simulink model "Ejercicio"  (R2023b)
settings: Solver=VariableStepAuto  StartTime=0.0  StopTime=100  RelTol=1e-3
settings Model: Creator=20808  LastModifiedBy=20808

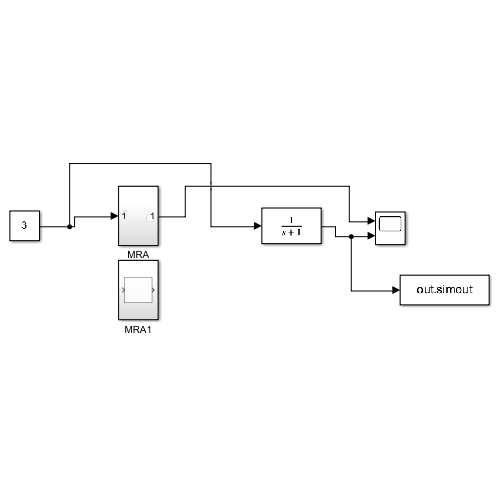
[thumbnail: Simulink's stored preview of the top-level diagram]
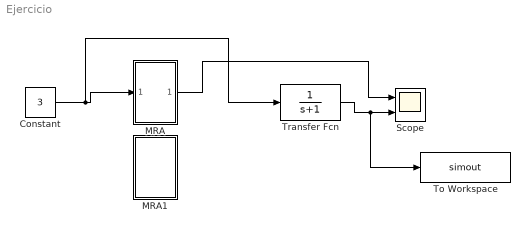
== system Ejercicio ==
  Constant : Constant  Value=3
  MRA : Subsystem
  MRA1 : Subsystem
  Scope : Scope  NumInputPorts=2
  To Workspace : ToWorkspace  VariableName=simout  SampleTime=-1
  Transfer Fcn : TransferFcn  Denominator=[1 1]
  wires:
  Constant/1 -> Transfer Fcn/1, MRA/1(In1)
  MRA/1(Out1) -> Scope/1
  Transfer Fcn/1 -> To Workspace/1, Scope/2

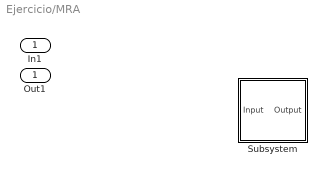
== system Ejercicio/MRA ==
  In1 : Inport
  Subsystem : Subsystem
  Out1 : Outport

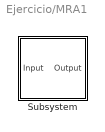
== system Ejercicio/MRA1 ==
  Subsystem : Subsystem

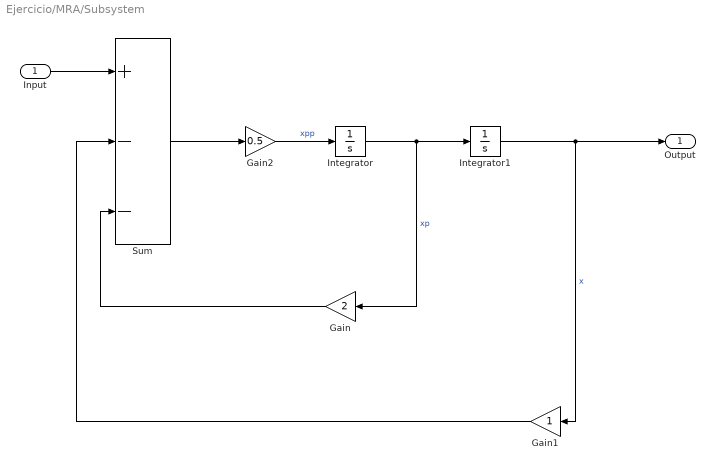
== system Ejercicio/MRA/Subsystem ==
  Input : Inport
  Gain : Gain  Gain=2
  Gain1 : Gain
  Gain2 : Gain  Gain=0.5
  Integrator : Integrator
  Integrator1 : Integrator
  Sum : Sum  Inputs=+--
  Output : Outport
  wires:
  Gain2/1 -> Integrator/1  "xpp"
  Sum/1 -> Gain2/1
  Integrator1/1 -> Output/1, Gain1/1  "x"
  Gain/1 -> Sum/3
  Input/1 -> Sum/1
  Gain1/1 -> Sum/2
  Integrator/1 -> Gain/1, Integrator1/1  "xp"

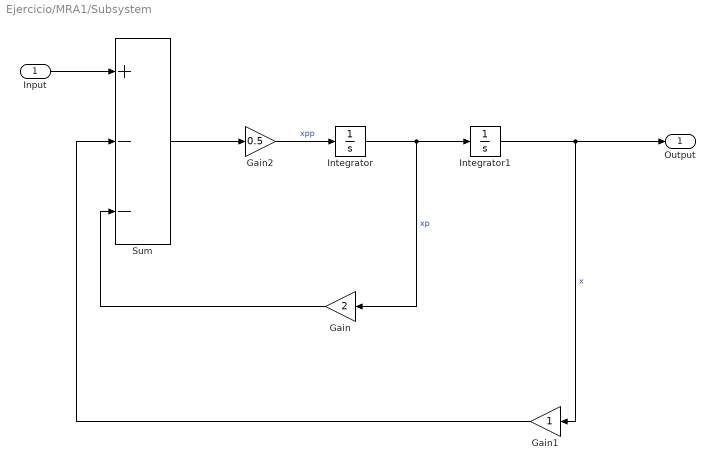
== system Ejercicio/MRA1/Subsystem ==
  Input : Inport
  Gain : Gain  Gain=2
  Gain1 : Gain
  Gain2 : Gain  Gain=0.5
  Integrator : Integrator
  Integrator1 : Integrator
  Sum : Sum  Inputs=+--
  Output : Outport
  wires:
  Gain2/1 -> Integrator/1  "xpp"
  Sum/1 -> Gain2/1
  Integrator1/1 -> Output/1, Gain1/1  "x"
  Gain/1 -> Sum/3
  Input/1 -> Sum/1
  Gain1/1 -> Sum/2
  Integrator/1 -> Gain/1, Integrator1/1  "xp"
